simulink model "kyvadloLQ"  (R2018a)
settings: Solver=FixedStepAuto  StartTime=0.0  StopTime=10  FixedStep=Ts  MaxStep=0.01  RelTol=1e-3  EnableMultiTasking=on
PreLoadFcn:
  | m1=0.4;        % Hmotnost vozika [kg]
  | m2=0.08;      % Hmotnost kyvadla [kg]
  | l=0.2;            % Vzdialenost taziska od osi rotacie [m]
  | g=9.81;         % Tiazove zrychlenie [m/s2]
  | b=0.1;           % Koeficient trenia [m/s]
StartFcn:
  | kyvadloOfflineLQ
values from neighbouring files (symbols this model uses):
  Klq = dlqr(A,B,Qlq,Rlq)    [kyvadloOfflineLQ.m]
  Ts = 5    [integrator.m]    (also in kyvadloOfflineLQ.m = kyvadlo.Ts; kyvadloOfflineMPC.m = kyvadlo.Ts; kyvadloOfflineMPCaKF.m = kyvadlo.Ts; stavovyprikaz.m = 0.5)
  uh = 0.002    [.m]    (also in MPCjedenkrok.m = 0.01; MPCuzavretaslucka.m = 0.01; integrator.m = 10; kombinovaneobmedzenia.m = 0.005)
  ul = -uh    (= -0.01)    [MPCjedenkrok.m]    (also in MPCuzavretaslucka.m; integrator.m = 0; kyvadloOfflineLQ.m = -5; kyvadloOfflineMPC.m = -5)
  x1h = 0.5    [kyvadloOfflineLQ.m]    (also in kyvadloOfflineMPC.m; kyvadloOfflineMPCaKF.m)
  x1l = -x1h    (= -0.5)    [kyvadloOfflineLQ.m]    (also in kyvadloOfflineMPC.m; kyvadloOfflineMPCaKF.m)
libraries: simulink x1
settings Model: Creator=UAMAI-LENOVO  LastModifiedBy=Gergely
settings DataIOCC: LimitDataPoints=on  SaveFormat=Array
settings OptimizationCC: LifeSpan=inf
settings DebuggingCC: SFUnexpectedBacktrackingDiag=warning  SFNoUnconditionalDefaultTransitionDiag=warning  SFExecutionAtInitializationDiag=none
settings HardwareCC: ProdBitPerPointer=32  ProdBitPerSizeT=32  ProdBitPerPtrDiffT=32  ProdLargestAtomicFloat=None  ProdIntDivRoundTo=Undefined  ProdEndianess=Unspecified  ProdWordSize=32  ProdHWDeviceType=32-bit Generic
settings ModelReferenceCC: PropagateSignalLabelsOutOfModel=off
settings CodeAppCC: StateflowObjectComments=on
settings GRTTargetCC: TargetLangStandard=C89/C90 (ANSI)  GeneratePreprocessorConditionals=Disable all
settings ConfigComp: CovMetricSettings=dw  CovHtmlReporting=on  CovSaveCumulativeToWorkspaceVar=on  CovSaveSingleToWorkspaceVar=on  CovExternalEMLEnable=off

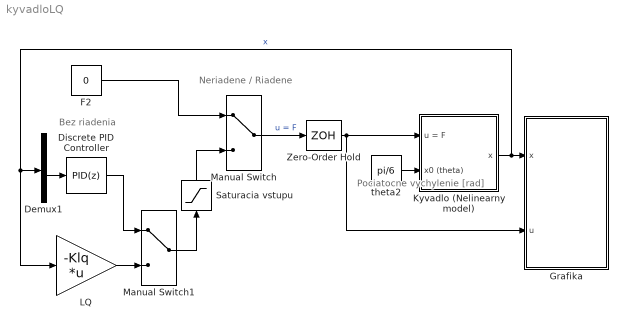
== system kyvadloLQ ==
  note: Pociatocne
      | vychylenie [rad]
  note: Neriadene / Riadene
  note: Bez riadenia
  Demux1 : Demux
  Discrete PID Controller : simulink/Continuous/PID Controller  Controller=PID  TimeDomain=Discrete-time  SampleTime=-1  IntegratorMethod=Forward Euler  FilterMethod=Forward Euler  Form=Parallel  UseFilter=on  ControllerParametersSource=internal  P=67.9471069093209  I=210.813906133692  D=4.71233666429646  N=193.181442099535  InitialConditionSource=internal  InitialConditionForIntegrator=0  InitialConditionForFilter=0  ExternalReset=none  LimitOutput=off  UpperSaturationLimit=inf  LowerSaturationLimit=-inf  LinearizeAsGain=off  AntiWindupMode=none  Kb=1  TrackingMode=off  Kt=1  PParamMin=[]  PParamMax=[]  IParamMin=[]  IParamMax=[]  DParamMin=[]  DParamMax=[]  NParamMin=[]  NParamMax=[]  KbParamMin=[]  KbParamMax=[]  KtParamMin=[]  KtParamMax=[]  POutMin=[]  POutMax=[]  IOutMin=[]  IOutMax=[]  DOutMin=[]  DOutMax=[]  NOutMin=[]  NOutMax=[]  KbOutMin=[]  KbOutMax=[]  KtOutMin=[]  KtOutMax=[]  IntegratorOutMin=[]  IntegratorOutMax=[]  FilterOutMin=[]  FilterOutMax=[]  SumOutMin=[]  SumOutMax=[]  SumI1OutMin=[]  SumI1OutMax=[]  SumI2OutMin=[]  SumI2OutMax=[]  SumI3OutMin=[]  SumI3OutMax=[]  SumDOutMin=[]  SumDOutMax=[]  SaturationOutMin=[]  SaturationOutMax=[]  IntegratorContinuousStateAttributes=''  IntegratorStateMustResolveToSignalObject=off  IntegratorRTWStateStorageClass=Auto  FilterContinuousStateAttributes=''  FilterStateMustResolveToSignalObject=off  FilterRTWStateStorageClass=Auto  DifferentiatorICPrevScaledInput=0  DifferentiatorOutMin=[]  DifferentiatorOutMax=[]  FilterDiffOutCoefMin=[]  FilterDiffOutCoefMax=[]  SumDenOutMin=[]  SumDenOutMax=[]  SumNumOutMin=[]  SumNumOutMax=[]  ReciprocalOutMin=[]  ReciprocalOutMax=[]  DivideOutMin=[]  DivideOutMax=[]  TunerSelectOption=Transfer Function Based (PID Tuner App)
  F2 : Constant  Value=0
  Grafika : Subsystem
  Kyvadlo (Nelinearny model) : Subsystem
  LQ : Gain  Gain=-Klq  Multiplication=Matrix(K*u) (u vector)
  Manual Switch : ManualSwitch
  Manual Switch1 : ManualSwitch
  Saturacia vstupu : Saturate  UpperLimit=uh  LowerLimit=ul
  Zero-Order Hold : ZeroOrderHold  SampleTime=Ts
  theta2 : Constant  Value=pi/6
  wires:
  F2/1 -> Manual Switch/1
  theta2/1 -> Kyvadlo (Nelinearny model)/2(x0 (theta))
  Kyvadlo (Nelinearny model)/1(x) -> LQ/1, Demux1/1, Grafika/1(x)  "x"
  Zero-Order Hold/1 -> Grafika/2(u), Kyvadlo (Nelinearny model)/1(u = F)
  Manual Switch/1 -> Zero-Order Hold/1  "u = F"
  LQ/1 -> Manual Switch1/2
  Saturacia vstupu/1 -> Manual Switch/2
  Manual Switch1/1 -> Saturacia vstupu/1
  Discrete PID Controller/1 -> Manual Switch1/1
  Demux1/3 -> Discrete PID Controller/1

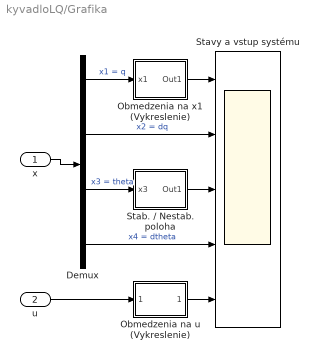
== system kyvadloLQ/Grafika ==
  x : Inport
  u : Inport  Port=2
  " Stavy a vstup systému" : Scope  NumInputPorts=5
  Demux : Demux
  Obmedzenia na u (Vykreslenie) : Subsystem
  "Obmedzenia na x1 (Vykreslenie) " : Subsystem
  Stab. / Nestab. poloha : Subsystem
  wires:
  Demux/2 -> " Stavy a vstup systému"/2  "x2 = dq"
  Demux/3 -> Stab. / Nestab. poloha/1(x3)  "x3 = theta"
  "Obmedzenia na x1 (Vykreslenie) "/1(Out1) -> " Stavy a vstup systému"/1
  u/1 -> Obmedzenia na u (Vykreslenie)/1(u = F)
  Demux/1 -> "Obmedzenia na x1 (Vykreslenie) "/1(x1)  "x1 = q"
  x/1 -> Demux/1
  Demux/4 -> " Stavy a vstup systému"/4  "x4 = dtheta"
  Stab. / Nestab. poloha/1(Out1) -> " Stavy a vstup systému"/3
  Obmedzenia na u (Vykreslenie)/1(Out1) -> " Stavy a vstup systému"/5

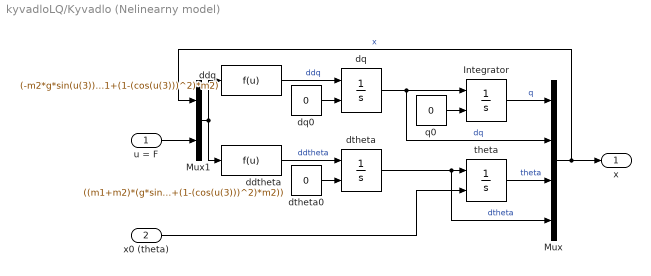
== system kyvadloLQ/Kyvadlo (Nelinearny model) ==
  u = F : Inport
  x0 (theta) : Inport  Port=2
  Integrator : Integrator  InitialConditionSource=external
  Mux : Mux
  Mux1 : Mux  Inputs=2
  ddq : Fcn  Expr=(-m2*g*sin(u(3))*cos(u(3))+m2*l*((u(4))^2)*sin(u(3))+b*m2*u(4)*cos(u(3))+u(5))/(m1+(1-(cos(u(3)))^2)*m2)
  ddtheta : Fcn  Expr=((m1+m2)*(g*sin(u(3))-b*u(4))-(m2*l*((u(4))^2)*sin(u(3))+u(5))*cos(u(3)))/(l*(m1+(1-(cos(u(3)))^2)*m2))
  dq : Integrator  InitialConditionSource=external
  dq0 : Constant  Value=0
  dtheta : Integrator  InitialConditionSource=external
  dtheta0 : Constant  Value=0
  q0 : Constant  Value=0
  theta : Integrator  InitialConditionSource=external
  x : Outport
  wires:
  Mux/1 -> x/1, Mux1/1  "x"
  ddq/1 -> dq/1  "ddq"
  dq/1 -> Mux/2, Integrator/1  "dq"
  ddtheta/1 -> dtheta/1  "ddtheta"
  x0 (theta)/1 -> theta/2
  q0/1 -> Integrator/2
  Integrator/1 -> Mux/1  "q"
  theta/1 -> Mux/3  "theta"
  dtheta/1 -> Mux/4, theta/1  "dtheta"
  Mux1/1 -> ddtheta/1, ddq/1
  dq0/1 -> dq/2
  dtheta0/1 -> dtheta/2
  u = F/1 -> Mux1/2

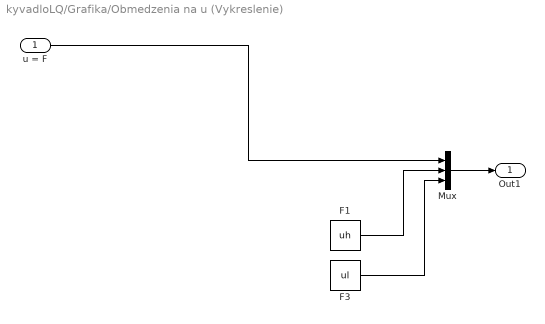
== system kyvadloLQ/Grafika/Obmedzenia na u (Vykreslenie) ==
  u = F : Inport
  F1 : Constant  Value=uh
  F3 : Constant  Value=ul
  Mux : Mux  Inputs=3
  Out1 : Outport
  wires:
  F1/1 -> Mux/2
  F3/1 -> Mux/3
  u = F/1 -> Mux/1
  Mux/1 -> Out1/1

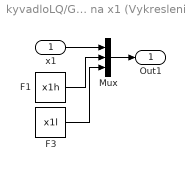
== system kyvadloLQ/Grafika/Obmedzenia na x1 (Vykreslenie)  ==
  x1 : Inport
  F1 : Constant  Value=x1h
  F3 : Constant  Value=x1l
  Mux : Mux  Inputs=3
  Out1 : Outport
  wires:
  F1/1 -> Mux/2
  F3/1 -> Mux/3
  x1/1 -> Mux/1
  Mux/1 -> Out1/1

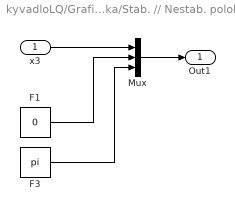
== system kyvadloLQ/Grafika/Stab. // Nestab. poloha ==
  x3 : Inport
  F1 : Constant  Value=0
  F3 : Constant  Value=pi
  Mux : Mux  Inputs=3
  Out1 : Outport
  wires:
  F1/1 -> Mux/2
  F3/1 -> Mux/3
  x3/1 -> Mux/1
  Mux/1 -> Out1/1
